simulink model "sixDOF_hw8"  (R2015a)
settings: Solver=ode8  StartTime=0.0  StopTime=t_total  FixedStep=dt  MaxStep=60  MinStep=.05  RelTol=1e-3
values from neighbouring files (symbols this model uses):
  A0 = zeros(3,3)    [PS2.m]    (also in PS3.m = getDCM(triad1, triad2); PS4.m = getDCM(triad1, triad2); PS5.m = getDCM(triad1, triad2); PS7.m = getDCM(triad1, triad2))
  a0 = 6776    [PS1.m]    (also in PS4.m; PS5.m; PS7.m)
  A_b2p = S_top.DCM_B2P    [PS5.m]    (also in PS7.m)
  b_perturbs = 1    [PS5.m]    (also in PS7.m; PS8.m; PS9.m)
  bControl = 1    [PS8.m]    (also in PS9.m)
  bGravGrad = 1    [PS1.m]    (also in PS4.m; PS5.m; PS7.m; PS8.m)
  bNoise = 1    [PS6.m]    (also in PS7.m; PS8.m = 0; PS9.m = 0)
  dt = 0.5    [PS8.m]    (also in PS9.m)
  e0 = 0.0004758    [PS1.m]    (also in PS4.m; PS5.m; PS7.m)
  H0 = eye(3)    [PS7.m]
  I_principle = S_top.tauCM_P    [PS2.m]    (also in PS3.m; PS4.m; PS5.m; PS7.m)
  incl0 = 51.6397    [PS1.m]    (also in PS4.m = 0; PS5.m = 0; PS7.m = 0)
  J2 = 0    [PS1.m]    (also in PS4.m; PS5.m; PS7.m)
  M0 = [0 0 0]'    [PS2.m]    (also in PS3.m; PS4.m; PS5.m; PS7.m)
  mu = 3.986e14 / 1000^3    (= 398600)    [PS1.m]    (also in PS4.m; PS5.m; PS7.m)
  normalsList = [normalsList, chd.normals]    [S_top2Lists.m]
  nu0 = 0    [PS1.m]    (also in PS4.m; PS5.m; PS7.m)
  OMEGA0 = 106.0758    [PS1.m]    (also in PS4.m = 0; PS5.m = 0; PS7.m = 0)
  omega0 = 233.6745    [PS1.m]    (also in PS4.m = 0; PS5.m = 0; PS7.m = 0)
  P0 = 0.01*eye(3)    [PS7.m]
  Q0 = P0 ./ 10    [PS7.m]
  R0 = (10 /180*pi)^2 * eye(3,3)    [PS7.m]
  Re = 6371    [PS1.m]    (also in PS4.m; PS5.m; PS7.m)
  surfaceAreasList = [surfaceAreasList; chd.surfaceAreas]    [S_top2Lists.m]
  surfaceCM_bodyList = [surfaceCM_bodyList, chd.surfaceCM_body]    [S_top2Lists.m]
  tOffset = 0    [PS5.m]    (also in PS7.m)
  UTC_0 = [06,02,2017]    [PS5.m]    (also in PS7.m)
  w0 = w0_28    [PS2.m]    (also in PS3.m = [0; 0; 10/180*pi*rand()]; PS4.m = w0 + 0.0007*[1 1 1]'; PS5.m = [0 -n0 0]'; PS7.m = [0 -2 0]')
  w_des = [0 -n0 0]'    [PS8.m]    (also in PS9.m = [0 0 0]')
  wEarth = [0 0 7.292116e-5]'    [PS5.m]    (also in PS7.m)
  x0 = rand(3,1)    [PS7.m]
undefined symbols (not defined in the file or in its folder): A_CMG0, Lw, u0
settings Model: Creator=Toby  LastModifiedBy=Toby
settings DataIOCC: SaveTime=off

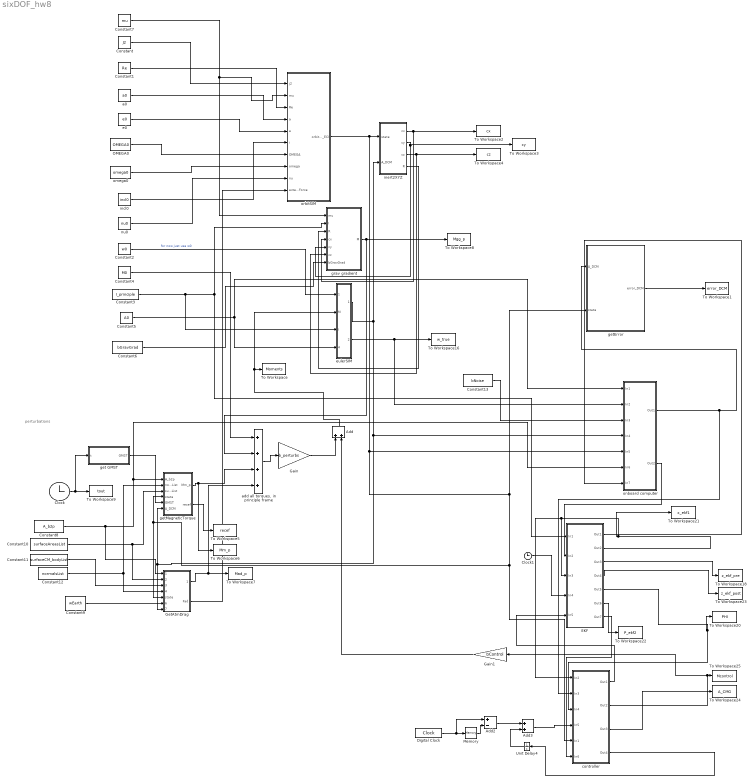
== system sixDOF_hw8 ==
  note: perturbations
  Add : Sum
  Add2 : Sum  Inputs=+-
  Add3 : Sum
  Clock : Clock
  Clock1 : Clock
  Constant : Constant  Value=J2
  Constant1 : Constant  Value=Re
  Constant10 : Constant  Value=surfaceAreasList
  Constant11 : Constant  Value=surfaceCM_bodyList
  Constant12 : Constant  Value=normalsList
  Constant13 : Constant  Value=bNoise
  Constant2 : Constant  Value=w0
  Constant3 : Constant  Value=I_principle
  Constant4 : Constant  Value=M0
  Constant5 : Constant  Value=A0
  Constant6 : Constant  Value=bGravGrad
  Constant7 : Constant  Value=mu
  Constant8 : Constant  Value=A_b2p
  Constant9 : Constant  Value=wEarth
  Digital Clock : DigitalClock  SampleTime=dt
  EKF : Subsystem
  Gain : Gain  Gain=b_perturbs
  Gain1 : Gain  Gain=bControl
  GetAtmDrag : MATLAB Function  TreatAsAtomicUnit=on
  Memory : Memory
  OMEGA0 : Constant  Value=OMEGA0
  To Workspace : ToWorkspace  VariableName=Moments  SampleTime=-1
  To Workspace1 : ToWorkspace  VariableName=error_DCM  SampleTime=-1
  To Workspace16 : ToWorkspace  VariableName=w_true  SampleTime=-1
  To Workspace18 : ToWorkspace  VariableName=z_ekf_pre  SampleTime=-1
  To Workspace2 : ToWorkspace  VariableName=cx  SampleTime=-1
  To Workspace20 : ToWorkspace  VariableName=PHI  SampleTime=-1
  To Workspace21 : ToWorkspace  VariableName=x_ekf1  SampleTime=-1
  To Workspace22 : ToWorkspace  VariableName=P_ekf2  SampleTime=-1
  To Workspace23 : ToWorkspace  VariableName=z_ekf_post  SampleTime=-1
  To Workspace24 : ToWorkspace  VariableName=A_CMG  SampleTime=-1
  To Workspace25 : ToWorkspace  VariableName=Mcontrol  SampleTime=-1
  To Workspace3 : ToWorkspace  VariableName=cy  SampleTime=-1
  To Workspace4 : ToWorkspace  VariableName=cz  SampleTime=-1
  To Workspace5 : ToWorkspace  VariableName=recef  SampleTime=-1
  To Workspace6 : ToWorkspace  VariableName=Mm_p  SampleTime=-1
  To Workspace7 : ToWorkspace  VariableName=Mad_p  SampleTime=-1
  To Workspace8 : ToWorkspace  VariableName=Mgg_p  SampleTime=-1
  To Workspace9 : ToWorkspace  VariableName=tout  SampleTime=-1
  Unit Delay4 : UnitDelay  InitialCondition=-50  SampleTime=-1
  a0 : Constant  Value=a0
  "add all torques, in principle frame" : Sum  Inputs=++++
  controller : Subsystem
  e0 : Constant  Value=e0
  eulerSIM : Subsystem
  get GMST : Subsystem
  getError : MATLAB Function  TreatAsAtomicUnit=on
  getMagneticTorque : MATLAB Function  TreatAsAtomicUnit=on
  grav gradient : MATLAB Function  TreatAsAtomicUnit=on
  incl0 : Constant  Value=incl0
  inert2XYZ : MATLAB Function  TreatAsAtomicUnit=on
  nu0 : Constant  Value=nu0
  omega0 : Constant  Value=omega0
  onboard computer : Subsystem
  orbitSIM : Subsystem
  wires:
  Constant7/1 -> grav gradient/1(mu), orbitSIM/2(mu)
  Constant/1 -> orbitSIM/1(j2)
  Constant1/1 -> orbitSIM/3(Re)
  a0/1 -> orbitSIM/4(a)
  e0/1 -> orbitSIM/5(e)
  OMEGA0/1 -> orbitSIM/7(OMEGA)
  omega0/1 -> orbitSIM/8(omega)
  incl0/1 -> orbitSIM/6(i)
  nu0/1 -> orbitSIM/9(nu)
  Constant5/1 -> onboard computer/1(In1), eulerSIM/4(A0)
  inert2XYZ/1(cx) -> grav gradient/4(cx), To Workspace2/1
  inert2XYZ/2(cy) -> To Workspace3/1, grav gradient/5(cy)
  inert2XYZ/4(R) -> grav gradient/3(R)
  inert2XYZ/3(cz) -> To Workspace4/1, grav gradient/6(cz)
  Constant6/1 -> grav gradient/7(bGravGrad)
  Add/1 -> eulerSIM/2(M), To Workspace/1
  GetAtmDrag/2(Fad) -> orbitSIM/10(externalForce)
  getError/1(error_DCM) -> To Workspace1/1
  grav gradient/1(M) -> "add all torques, in principle frame"/2, To Workspace8/1
  eulerSIM/1(A_DCM) -> inert2XYZ/2(A_DCM), getMagneticTorque/6(A_DCM), GetAtmDrag/7(A_DCM), onboard computer/4(In4)
  "add all torques, in principle frame"/1 -> Gain/1
  Clock/1 -> get GMST/1(t), To Workspace9/1
  Constant8/1 -> onboard computer/6(In6), getMagneticTorque/1(A_b2p), GetAtmDrag/1(A_b2p)
  GetAtmDrag/1(Mad_p) -> To Workspace7/1, "add all torques, in principle frame"/4
  Constant9/1 -> GetAtmDrag/6(wEarth)
  get GMST/1(GMST) -> getMagneticTorque/5(GMST)
  getMagneticTorque/2(recef) -> To Workspace5/1
  getMagneticTorque/1(Mm_p) -> "add all torques, in principle frame"/3, To Workspace6/1
  Constant12/1 -> getMagneticTorque/2(normalsList), GetAtmDrag/4(normalsList)
  Constant11/1 -> GetAtmDrag/3(surfaceCM_bodyList)
  Constant10/1 -> getMagneticTorque/3(surfaceAreasList), GetAtmDrag/2(surfaceAreasList)
  Constant4/1 -> "add all torques, in principle frame"/1
  eulerSIM/2(w_true) -> onboard computer/2(In2), To Workspace16/1
  Constant3/1 -> EKF/1(In1), grav gradient/2(I), eulerSIM/3(I)
  Constant2/1 -> eulerSIM/1(w0)  "for now just use w0"
  Gain/1 -> Add/1
  Gain1/1 -> Add/2
  Digital Clock/1 -> Add2/1, Memory/1
  Memory/1 -> Add2/2
  Add2/1 -> Add3/1
  Unit Delay4/1 -> Add3/2
  Constant13/1 -> onboard computer/3(In3)
  EKF/2(Out2) -> controller/1(In2), EKF/3(In3), To Workspace21/1
  EKF/5(Out5) -> To Workspace20/1, controller/3(In4)
  onboard computer/2(Out2) -> EKF/2(In2)
  Clock1/1 -> EKF/4(In4)
  EKF/1(Out1) -> onboard computer/7(In7)
  EKF/3(Out3) -> To Workspace18/1
  EKF/4(Out4) -> To Workspace23/1
  EKF/6(Out6) -> To Workspace22/1
  controller/2(Out2) -> Gain1/1, To Workspace25/1
  Add3/1 -> controller/4(In5)
  controller/1(Out1) -> EKF/5(In5)
  controller/3(Out3) -> To Workspace24/1
  controller/4(Out4) -> Unit Delay4/1
  onboard computer/1(Out1) -> controller/2(In3), getError/1(A_DCM)
  orbitSIM/1(orbit_state_ECI) -> controller/5(In1), getMagneticTorque/4(state), GetAtmDrag/5(state), getError/2(state), onboard computer/5(In5), inert2XYZ/1(state)
  EKF/7(Out7) -> controller/6(In6)

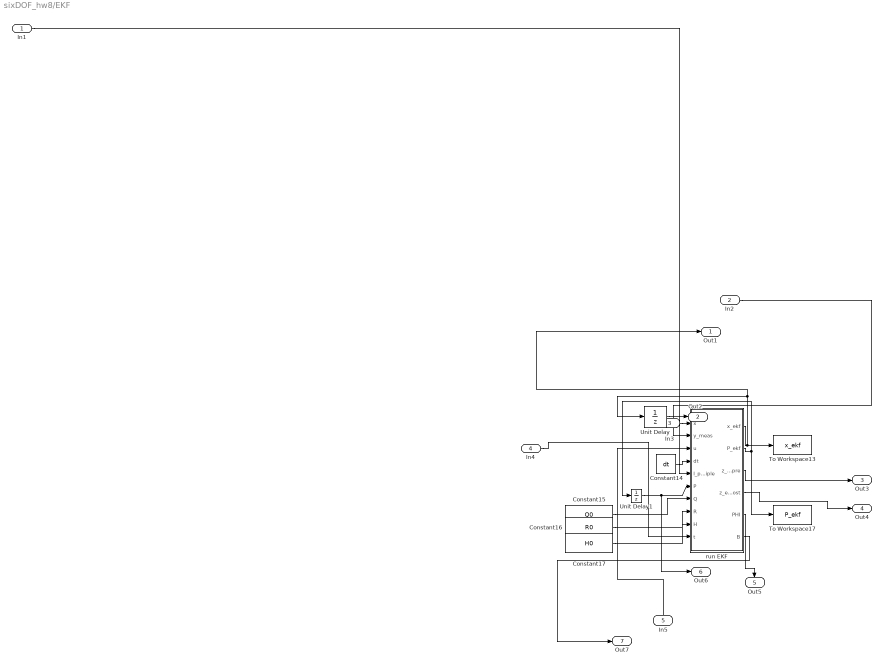
== system sixDOF_hw8/EKF ==
  In1 : Inport
  In2 : Inport  Port=2
  In3 : Inport  Port=3
  In4 : Inport  Port=4
  In5 : Inport  Port=5
  Constant14 : Constant  Value=dt
  Constant15 : Constant  Value=Q0
  Constant16 : Constant  Value=R0
  Constant17 : Constant  Value=H0
  To Workspace13 : ToWorkspace  VariableName=x_ekf  SampleTime=-1
  To Workspace17 : ToWorkspace  VariableName=P_ekf  SampleTime=-1
  Unit Delay : UnitDelay  InitialCondition=x0  SampleTime=-1
  Unit Delay1 : UnitDelay  InitialCondition=P0  SampleTime=-1
  run EKF : MATLAB Function  TreatAsAtomicUnit=on
  Out1 : Outport
  Out2 : Outport  Port=2
  Out3 : Outport  Port=3
  Out4 : Outport  Port=4
  Out5 : Outport  Port=5
  Out6 : Outport  Port=6
  Out7 : Outport  Port=7
  wires:
  Constant17/1 -> run EKF/9(H)
  run EKF/2(P_ekf) -> To Workspace17/1, Unit Delay1/1
  Unit Delay1/1 -> Out6/1, run EKF/6(P)
  Constant16/1 -> run EKF/8(R)
  Constant15/1 -> run EKF/7(Q)
  run EKF/6(B) -> Out7/1
  run EKF/4(z_ekf_post) -> Out4/1
  run EKF/3(z_ekf_pre) -> Out3/1
  In4/1 -> run EKF/10(t)
  run EKF/1(x_ekf) -> To Workspace13/1, Out1/1, Unit Delay/1
  run EKF/5(PHI) -> Out5/1
  Constant14/1 -> run EKF/4(dt)
  Unit Delay/1 -> Out2/1
  In1/1 -> run EKF/5(I_principle)
  In3/1 -> run EKF/1(x)
  In2/1 -> run EKF/2(y_meas)
  In5/1 -> run EKF/3(u)

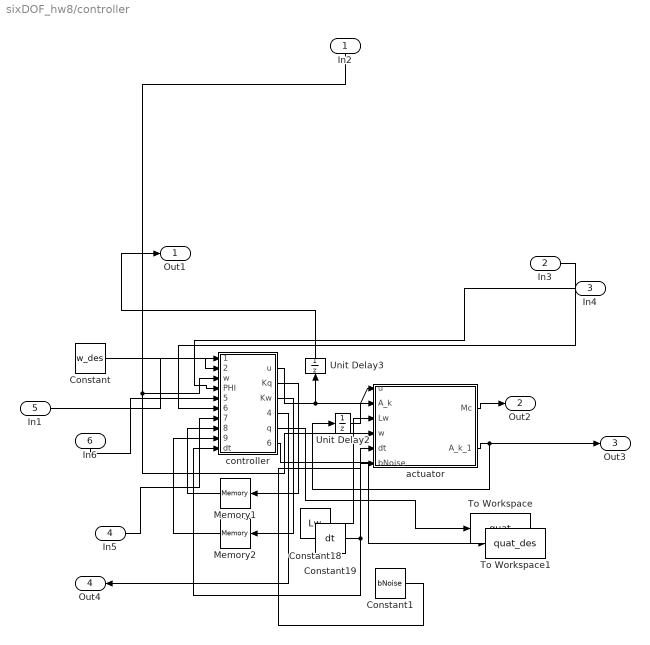
== system sixDOF_hw8/controller ==
  In2 : Inport
  In3 : Inport  Port=2
  In4 : Inport  Port=3
  In5 : Inport  Port=4
  In1 : Inport  Port=5
  In6 : Inport  Port=6
  Constant : Constant  Value=w_des
  Constant1 : Constant  Value=bNoise
  Constant18 : Constant  Value=Lw
  Constant19 : Constant  Value=dt
  Memory1 : Memory  X0=zeros(4)
  Memory2 : Memory  X0=zeros(3)
  To Workspace : ToWorkspace  VariableName=quat  SampleTime=-1
  To Workspace1 : ToWorkspace  VariableName=quat_des  SampleTime=-1
  Unit Delay2 : UnitDelay  InitialCondition=A_CMG0  SampleTime=-1
  Unit Delay3 : UnitDelay  InitialCondition=u0  SampleTime=-1
  actuator : MATLAB Function  TreatAsAtomicUnit=on
  controller : MATLAB Function  TreatAsAtomicUnit=on
  Out1 : Outport
  Out2 : Outport  Port=2
  Out3 : Outport  Port=3
  Out4 : Outport  Port=4
  wires:
  In5/1 -> controller/7(timePass)
  controller/2(Kq) -> Memory1/1
  Memory1/1 -> controller/8(Kq_old)
  controller/4(timePass1) -> Out4/1
  actuator/1(Mc) -> Out2/1
  Constant18/1 -> actuator/3(Lw)
  controller/1(u) -> Unit Delay3/1, actuator/1(u)
  Unit Delay2/1 -> actuator/2(A_k)
  actuator/2(A_k_1) -> Out3/1, Unit Delay2/1
  Constant19/1 -> actuator/5(dt), controller/10(dt)
  In3/1 -> controller/6(A_DCM)
  Unit Delay3/1 -> Out1/1
  In2/1 -> controller/3(w), actuator/4(w)
  In4/1 -> controller/4(PHI)
  Constant/1 -> controller/2(w_des)
  In1/1 -> controller/1(state)
  In6/1 -> controller/5(Beuler)
  controller/3(Kw) -> Memory2/1
  Memory2/1 -> controller/9(Kw_old)
  controller/5(q) -> To Workspace/1
  controller/6(q_des) -> To Workspace1/1
  Constant1/1 -> actuator/6(bNoise)

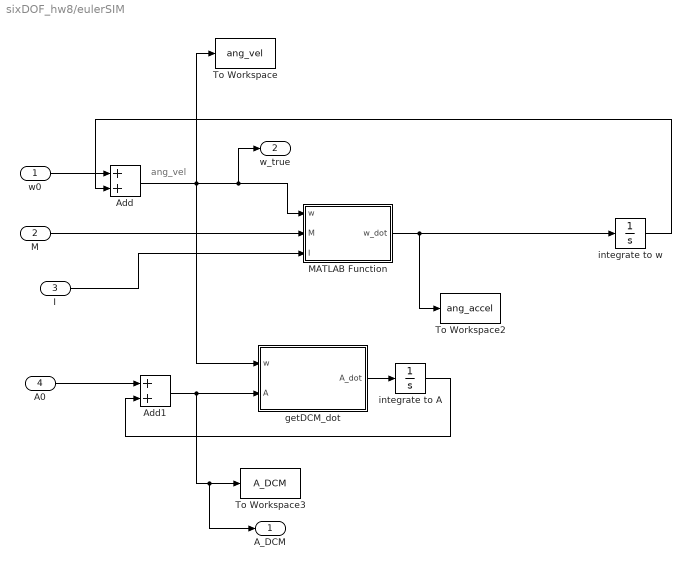
== system sixDOF_hw8/eulerSIM ==
  note: ang_vel
  w0 : Inport
  M : Inport  Port=2
  I : Inport  Port=3
  A0 : Inport  Port=4
  Add : Sum
  Add1 : Sum
  MATLAB Function : MATLAB Function  TreatAsAtomicUnit=on
  To Workspace : ToWorkspace  VariableName=ang_vel  SampleTime=-1
  To Workspace2 : ToWorkspace  VariableName=ang_accel  SampleTime=-1
  To Workspace3 : ToWorkspace  VariableName=A_DCM  SampleTime=-1
  getDCM_dot : MATLAB Function  TreatAsAtomicUnit=on
  integrate to A : Integrator
  integrate to w : Integrator
  A_DCM : Outport
  w_true : Outport  Port=2
  wires:
  w0/1 -> Add/1
  M/1 -> MATLAB Function/2(M)
  Add1/1 -> A_DCM/1, To Workspace3/1, getDCM_dot/2(A)
  I/1 -> MATLAB Function/3(I)
  getDCM_dot/1(A_dot) -> integrate to A/1
  A0/1 -> Add1/1
  integrate to A/1 -> Add1/2
  MATLAB Function/1(w_dot) -> integrate to w/1, To Workspace2/1
  integrate to w/1 -> Add/2
  Add/1 -> getDCM_dot/1(w), To Workspace/1, w_true/1, MATLAB Function/1(w)

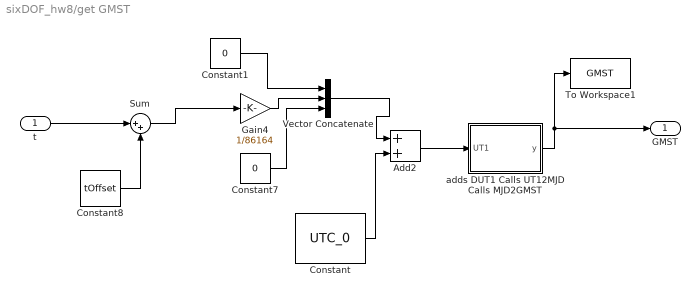
== system sixDOF_hw8/get GMST ==
  t : Inport
  Add2 : Sum
  Constant : Constant  Value=UTC_0
  Constant1 : Constant  Value=0
  Constant7 : Constant  Value=0
  Constant8 : Constant  Value=tOffset
  Gain4 : Gain  Gain=1/86164
  Sum : Sum  Inputs=|++
  To Workspace1 : ToWorkspace  VariableName=GMST  SampleTime=-1
  Vector Concatenate : Concatenate  NumInputs=3
  adds DUT1 Calls UT12MJD Calls MJD2GMST : MATLAB Function  TreatAsAtomicUnit=on
  GMST : Outport
  wires:
  Constant/1 -> Add2/2
  Constant7/1 -> Vector Concatenate/3
  Gain4/1 -> Vector Concatenate/2
  Constant1/1 -> Vector Concatenate/1
  Vector Concatenate/1 -> Add2/1
  Add2/1 -> adds DUT1 Calls UT12MJD Calls MJD2GMST/1(UT1)
  Sum/1 -> Gain4/1
  t/1 -> Sum/1
  Constant8/1 -> Sum/2
  adds DUT1 Calls UT12MJD Calls MJD2GMST/1(y) -> GMST/1, To Workspace1/1

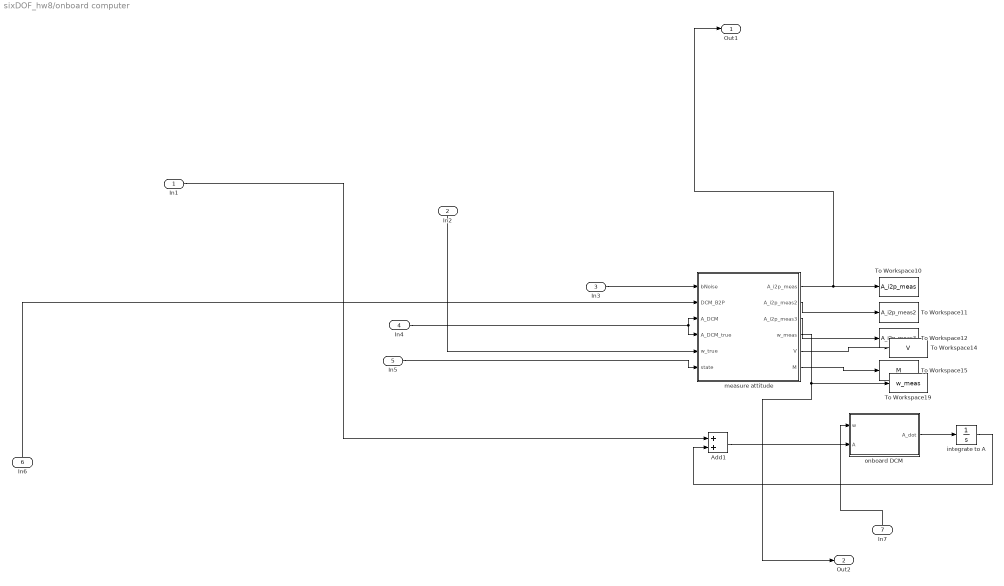
== system sixDOF_hw8/onboard computer ==
  In1 : Inport
  In2 : Inport  Port=2
  In3 : Inport  Port=3
  In4 : Inport  Port=4
  In5 : Inport  Port=5
  In6 : Inport  Port=6
  In7 : Inport  Port=7
  Add1 : Sum
  To Workspace10 : ToWorkspace  VariableName=A_i2p_meas  SampleTime=-1
  To Workspace11 : ToWorkspace  VariableName=A_i2p_meas2  SampleTime=-1
  To Workspace12 : ToWorkspace  VariableName=A_i2p_meas3  SampleTime=-1
  To Workspace14 : ToWorkspace  VariableName=V  SampleTime=-1
  To Workspace15 : ToWorkspace  VariableName=M  SampleTime=-1
  To Workspace19 : ToWorkspace  VariableName=w_meas  SampleTime=-1
  integrate to A : Integrator
  measure attitude : MATLAB Function  TreatAsAtomicUnit=on
  onboard DCM : MATLAB Function  TreatAsAtomicUnit=on
  Out1 : Outport
  Out2 : Outport  Port=2
  wires:
  In4/1 -> measure attitude/4(A_DCM_true), measure attitude/3(A_DCM)
  In5/1 -> measure attitude/6(state)
  In6/1 -> measure attitude/2(DCM_B2P)
  In2/1 -> measure attitude/5(w_true)
  In1/1 -> Add1/1
  In7/1 -> onboard DCM/1(w)
  Add1/1 -> onboard DCM/2(A)
  measure attitude/3(A_i2p_meas3) -> To Workspace12/1
  measure attitude/2(A_i2p_meas2) -> To Workspace11/1
  measure attitude/1(A_i2p_meas) -> Out1/1, To Workspace10/1
  measure attitude/4(w_meas) -> Out2/1, To Workspace19/1
  In3/1 -> measure attitude/1(bNoise)
  measure attitude/5(V) -> To Workspace14/1
  integrate to A/1 -> Add1/2
  onboard DCM/1(A_dot) -> integrate to A/1
  measure attitude/6(M) -> To Workspace15/1

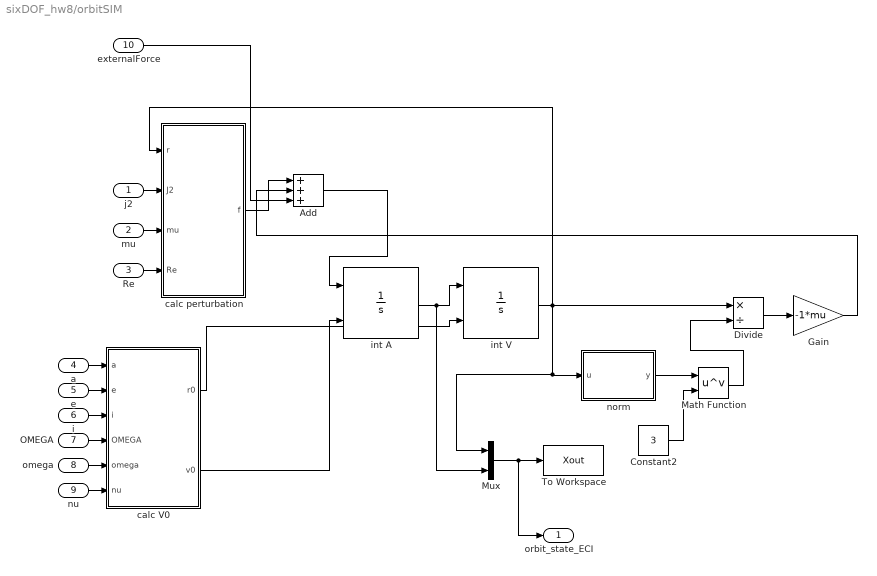
== system sixDOF_hw8/orbitSIM ==
  j2 : Inport
  mu : Inport  Port=2
  Re : Inport  Port=3
  a : Inport  Port=4
  e : Inport  Port=5
  i : Inport  Port=6
  OMEGA : Inport  Port=7
  omega : Inport  Port=8
  nu : Inport  Port=9
  externalForce : Inport  Port=10
  Add : Sum  Inputs=+++
  Constant2 : Constant  Value=3
  Divide : Product  Inputs=*/
  Gain : Gain  Gain=-1*mu
  Math Function : Math  Operator=pow  SaturateOnIntegerOverflow=on
  Mux : Mux  Inputs=2
  To Workspace : ToWorkspace  VariableName=Xout  SampleTime=-1
  calc V0 : MATLAB Function  TreatAsAtomicUnit=on
  calc perturbation : MATLAB Function  TreatAsAtomicUnit=on
  int A : Integrator  InitialConditionSource=external
  int V : Integrator  InitialConditionSource=external
  norm : MATLAB Function  TreatAsAtomicUnit=on
  orbit_state_ECI : Outport
  wires:
  calc V0/1(r0) -> int V/2
  Add/1 -> int A/1
  Mux/1 -> orbit_state_ECI/1, To Workspace/1
  norm/1(y) -> Math Function/1
  int V/1 -> calc perturbation/1(r), norm/1(u), Mux/1, Divide/1
  Math Function/1 -> Divide/2
  Divide/1 -> Gain/1
  Gain/1 -> Add/2
  calc V0/2(v0) -> int A/2
  int A/1 -> Mux/2, int V/1
  calc perturbation/1(f) -> Add/1
  Constant2/1 -> Math Function/2
  e/1 -> calc V0/2(e)
  i/1 -> calc V0/3(i)
  OMEGA/1 -> calc V0/4(OMEGA)
  a/1 -> calc V0/1(a)
  Re/1 -> calc perturbation/4(Re)
  mu/1 -> calc perturbation/3(mu)
  omega/1 -> calc V0/5(omega)
  j2/1 -> calc perturbation/2(J2)
  nu/1 -> calc V0/6(nu)
  externalForce/1 -> Add/3

== matlab function sixDOF_hw8/orbitSIM/norm ==
  data: u input; y output
function y = fcn(u)
%#codegen

y = norm(u);

== matlab function sixDOF_hw8/orbitSIM/calc perturbation ==
  data: r input; f output; J2 input; mu input; Re input
function f = fcn(r, J2, mu, Re)
% NOTE! EVERYTHING IN DEGREES
% 
% fR = -3*mu*J2*Re^2/(2*r^4)*(1-3*sind(incl)^2*sind(u)^2);
% fT = -3*mu*J2*Re^2/(2*r^4)*(sind(incl)^2*sind(u)*cosd(u));
% fN = -3*mu*J2*Re^2/(2*r^4)*(sind(incl)*cosd(incl)*sind(u));
rMag = norm(r);
rDir = r ./ norm(r);
f = -mu*J2*Re^2/2*( [0, 0, 6*r(3)/rMag^5]' + ...
      (3/rMag^4 - 15*(r(3)^2/rMag^6)).*rDir);

end

== matlab function sixDOF_hw8/orbitSIM/calc V0 ==
  data: a input; r0 output; e input; i input; OMEGA input; omega input; nu input; v0 output
function [r0, v0] = fcn(a, e, i, OMEGA, omega, nu)
%#codegen
[r0, v0] = OE2XV(a, e, i, OMEGA, omega, nu);
end

== matlab function sixDOF_hw8/getMagneticTorque ==
  data: A_b2p input; Mm_p output; normalsList input; surfaceAreasList input; state input; GMST input; A_DCM input; recef output
function [Mm_p, recef] = fcn(A_b2p, normalsList, surfaceAreasList, state, GMST, A_DCM)
%#codegen

coder.extrinsic('magneticTorque'); 
xECI = state(1:3);
r = norm(xECI);
[ longitude, latitude, recef ] = getLongLatECEF( xECI, GMST );
Mm_p = [0 0 0]';
if false
  [ Mm_p ] = magneticTorque( A_b2p, surfaceAreasList, normalsList, ...
  longitude, latitude, r, A_DCM, GMST);
end
end

== matlab function sixDOF_hw8/GetAtmDrag ==
  data: A_b2p input; Mad_p output; surfaceAreasList input; surfaceCM_bodyList input; normalsList input; state input; wEarth input; A_DCM input; Fad output
function [Mad_p, Fad] = fcn(A_b2p, surfaceAreasList, surfaceCM_bodyList, ...
  normalsList, state, wEarth, A_DCM)
%#codegen
xECI = state(1:3);
V_sc = state(4:6);
[ Fad, Mad ] = atmDragTorque(A_b2p, surfaceAreasList, surfaceCM_bodyList, ...
    normalsList, xECI, A_DCM, wEarth, V_sc );
A_p2i = getP2IfromA_DCM(A_DCM);
Mad_p = A_p2i' * Mad;
end

== matlab function sixDOF_hw8/getError ==
  data: A_DCM input; error_DCM output; state input
function error_DCM = fcn(A_DCM, state)
%#codegen
[ error_DCM ] = getAttError( A_DCM, state);

== matlab function sixDOF_hw8/eulerSIM/MATLAB Function ==
  data: w input; w_dot output; M input; I input
function w_dot = eulerRHS(w, M, I)
% principle axis euler eq
% w is 3x1 rotational velocity, expressed in principle
% M is 3x1 external torques, expressed in principle
Ix = I(1,1); Iy = I(2,2); Iz = I(3,3);
w_dot = zeros(3,1);
w_dot(1) = (M(1) - (Iz - Iy)*w(2)*w(3) ) / Ix;
w_dot(2) = (M(2) - (Ix - Iz)*w(1)*w(3) ) / Iy;
w_dot(3) = (M(3) - (Iy - Ix)*w(1)*w(2) ) / Iz;
end

== matlab function sixDOF_hw8/eulerSIM/getDCM_dot ==
  data: w input; A_dot output; A input
function A_dot   = getDCM_dot( w, A )
%GETDCM_DOT calculate time-derivative of DCM
% w is ang vel of body axes w.r.t. inertial EXPRESSED IN INERTIAL
[ A_dot ] = getDCM_dot( w, A );

end

== matlab function sixDOF_hw8/grav gradient ==
  data: mu input; M output; I input; R input; cx input; cy input; cz input; bGravGrad input
function M = fcn(mu, I, R, cx, cy, cz, bGravGrad)
%#codegen
if bGravGrad
  M = gravGradient( mu, I, R, cx, cy, cz );
else
  M = [0 0 0]';
end

== matlab function sixDOF_hw8/inert2XYZ ==
  data: cx output; state input; A_DCM input; cy output; cz output; R output
function [cx, cy, cz, R] = fcn(state, A_DCM)
%#codegen
%A should be principle to inertial
A = getP2IfromA_DCM( A_DCM );
R = norm(state(1:3));
c = 1 / R * A' * state(1:3);
cx = c(1);
cy = c(2);
cz = c(3);

== matlab function sixDOF_hw8/get GMST/adds DUT1 Calls UT12MJD Calls MJD2GMST ==
  data: UT1 input; y output
function y = fcn(UT1)
%u is calendar form
% DUT1= (UT1-UTC) transmitted with time signals                         
%              =  +0.5 seconds beginning 26 Jan 2017 at 0000 UTC  
UT1(2) = UT1(2) + 0.5; %defined offset
y1 = UT12MJD(UT1);
y = MJD2GMST(y1);

end

== matlab function sixDOF_hw8/onboard computer/measure attitude ==
  data: bNoise input; DCM_B2P input; A_i2p_meas output; A_DCM input; A_DCM_true input; w_true input; state input; A_i2p_meas2 output; A_i2p_meas3 output; w_meas output; V output; M output
function [ A_i2p_meas, A_i2p_meas2, A_i2p_meas3, w_meas, V,M ] = fcn( bNoise, DCM_B2P, A_DCM, A_DCM_true, w_true, state )
%#codegen
[ A_i2p_meas, A_i2p_meas2, A_i2p_meas3, V, M ] = measureAtt( bNoise, DCM_B2P, A_DCM, A_DCM_true, state );
w_meas = measureOMEGA(w_true, DCM_B2P, bNoise);

== matlab function sixDOF_hw8/onboard computer/onboard DCM ==
  data: w input; A_dot output; A input
function A_dot   = getDCM_dot( w, A )
%GETDCM_DOT calculate time-derivative of DCM
% w is ang vel of body axes w.r.t. inertial EXPRESSED IN INERTIAL
[ A_dot ] = getDCM_dot( w, A );

end

== matlab function sixDOF_hw8/EKF/run EKF ==
  data: x input; y_meas input; u input; x_ekf output; dt input; I_principle input; P input; Q input; R input; H input; P_ekf output; z_ekf_pre output; z_ekf_post output; PHI output; t input; B output
function [x_ekf, P_ekf, z_ekf_pre, z_ekf_post, PHI, B] = fcn(x, y_meas, u, dt, I_principle, ...
  P, Q, R, H, t)
%#codegen
[ PHI, B ] = linearEuler( y_meas, dt, I_principle );
[ x_k, P_ekf, z_ekf_pre, z_ekf_post ] = EKF( x, y_meas, u, PHI, B, ...
            P, Q, R, H);
          
x_ekf = x_k;

== matlab function sixDOF_hw8/controller/controller ==
  data: state input; w_des input; w input; u output; PHI input; Beuler input; A_DCM input; timePass input; Kq output; Kw output; Kq_old input; Kw_old input; timePass1 output; dt input; q output; q_des output
function [u, Kq, Kw, timePass1, q, q_des]  = fcn(state, w_des, w, PHI, Beuler, A_DCM, timePass, Kq_old, Kw_old, dt)
%#codegen
% x = [quat; ang vel]

triad1 = getRTNTriadfromState( state );
A_RTN = getDCM(triad1, eye(3));
coder.extrinsic('DCM2Quat_3rdTry')
q_des = coder.nullcopy(zeros(4,1));
q = coder.nullcopy(zeros(4,1));
q_des = DCM2Quat_3rdTry(A_RTN);
q = DCM2Quat_3rdTry(A_DCM);

coder.extrinsic('dlqr')
coder.extrinsic('lqr')
if timePass > 50*dt
  [Aquat, Aee, Bquat] = linearQuat( q, w, dt, Beuler );
  A = dt*eye(4);
  B = [zeros(4,1), Aee];
  C = eye(4);
  p = 2;
  Q = p*(C'*C);
  R = eye(size(B,2));

  Kq = coder.nullcopy(zeros(4));
  Kq = dlqr(A,B,Q,R); %discrete lqr, x_k+1 = A*x_k+B*u_k
  out = -Kq*(q - q_des);
  w_des = out(2:4);
  
  A = PHI;
  B = Beuler;
  C = eye(3);
  p = 100;
  Q = p*(C'*C);
  R = eye(size(B,2));
  Kw = coder.nullcopy(zeros(3));
  Kw = dlqr(A,B,Q,R);
  u = -Kw*(w - w_des);
  
  
  
  
  timePass1 = 0;
else
  Kq = Kq_old;
  Kw = Kw_old;
  timePass1 = timePass;
end
out = -Kq*(q - q_des);
u = -Kw*(w - out(2:4));

== matlab function sixDOF_hw8/controller/actuator ==
  data: u input; Mc output; A_k_1 output; A_k input; Lw input; w input; dt input; bNoise input
function [Mc, A_k_1] = fcn(u, A_k, Lw, w, dt, bNoise)
%#codegen
% u = M_desired
Mc = zeros(3,1);
Mc(:) = u(:);
if bNoise
  Mc = Mc + 0.01*rand(3,1);
end
A_dot = 1/Lw*(-cross(w,A_k*Lw) - Mc);
%perfect, instantaneous actuators!
A_k_1 = A_k + dt*A_dot;
